simulink model "RCAM_simulation_trim_template"  (R2021b)
settings: Solver=VariableStepAuto  StartTime=0.0  StopTime=TF  RelTol=1e-3
values from neighbouring files (symbols this model uses):
  x0 = [75 ... (first row only)    [initializeConstants.m]
undefined symbols (not defined in the file or in its folder): RCAM_model
settings Model: Creator=khanh  LastModifiedBy=khanh

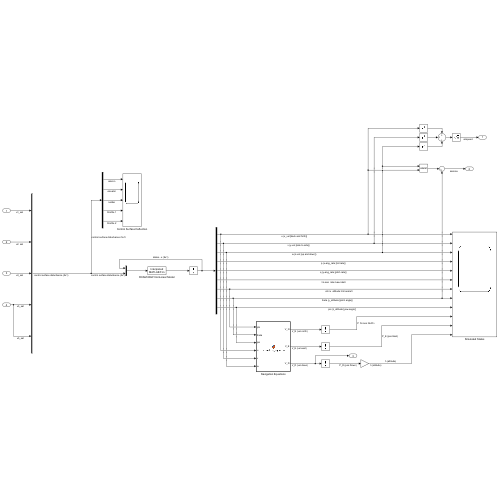
[thumbnail: Simulink's stored preview of the top-level diagram]
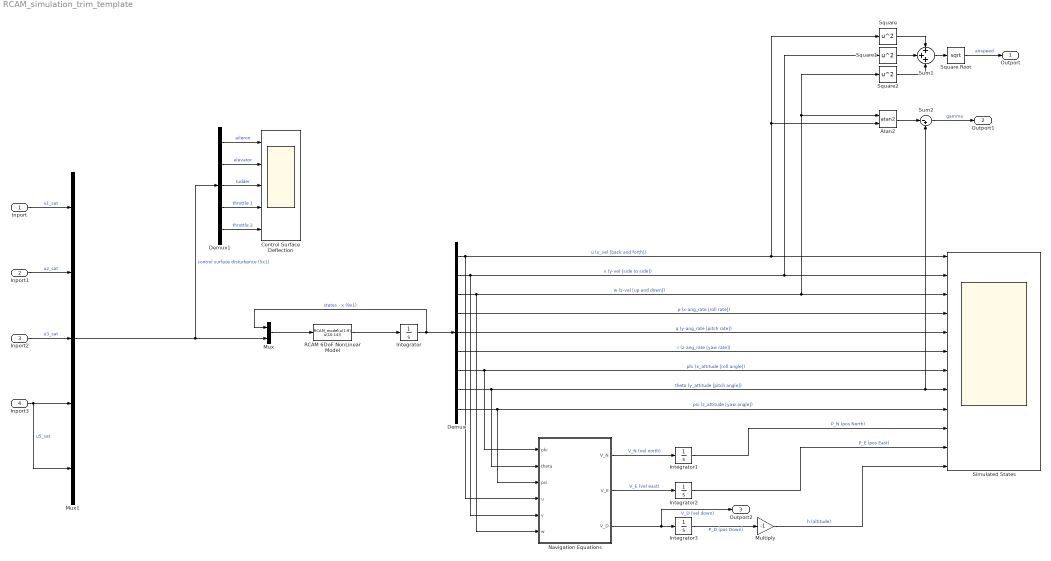
== system RCAM_simulation_trim_template ==
  Inport : Inport
  Inport1 : Inport  Port=2
  Inport2 : Inport  Port=3
  Inport3 : Inport  Port=4
  Atan2 : Trigonometry  Operator=atan2
  Control Surface Deflection : Scope  NumInputPorts=5
  Demux : Demux  Outputs=9
  Demux1 : Demux  Outputs=5
  Integrator : Integrator  InitialCondition=x0
  Integrator1 : Integrator  ContinuousStateAttributes='P_N'
  Integrator2 : Integrator  ContinuousStateAttributes='P_E'
  Integrator3 : Integrator  ContinuousStateAttributes='P_D'
  Multiply : Gain  Gain=-1
  Mux : Mux  Inputs=2
  Mux1 : Mux  Inputs=5
  Navigation Equations : MATLAB Function  TreatAsAtomicUnit=on
  RCAM 6DoF NonLinear Model : MATLABFcn  MATLABFcn=RCAM_model(u(1:9), u(10:14))
  Simulated States : Scope  NumInputPorts=12
  Square : Math  Operator=square  SaturateOnIntegerOverflow=on
  Square Root : Sqrt  SaturateOnIntegerOverflow=on
  Square1 : Math  Operator=square  SaturateOnIntegerOverflow=on
  Square2 : Math  Operator=square  SaturateOnIntegerOverflow=on
  Sum1 : Sum  Inputs=+++
  Sum2 : Sum  Inputs=|-+
  Outport : Outport
  Outport1 : Outport  Port=2
  Outport2 : Outport  Port=3
  wires:
  RCAM 6DoF NonLinear Model/1 -> Integrator/1
  Integrator/1 -> Demux/1, Mux/1  "states - x (9x1)"
  Mux/1 -> RCAM 6DoF NonLinear Model/1
  Inport/1 -> Mux1/1  "u1_sat"
  Inport3/1 -> Mux1/5, Mux1/4  "u5_sat"
  Inport2/1 -> Mux1/3  "u3_sat"
  Inport1/1 -> Mux1/2  "u2_sat"
  Demux1/1 -> Control Surface Deflection/1  "aileron"
  Demux1/2 -> Control Surface Deflection/2  "elevator"
  Demux1/3 -> Control Surface Deflection/3  "rudder"
  Demux1/4 -> Control Surface Deflection/4  "throttle 1"
  Demux1/5 -> Control Surface Deflection/5  "throttle 2"
  Mux1/1 -> Demux1/1, Mux/2  "control surface disturbance (5x1)"
  Demux/1 -> Navigation Equations/4(u), Atan2/2, Square/1, Simulated States/1  "u (x_vel [back and forth])"
  Demux/2 -> Navigation Equations/5(v), Square1/1, Simulated States/2  "v (y-vel [side to side])"
  Demux/3 -> Navigation Equations/6(w), Atan2/1, Square2/1, Simulated States/3  "w (z-vel [up and down])"
  Demux/4 -> Simulated States/4  "p (x-ang_rate [roll rate])"
  Demux/5 -> Simulated States/5  "q (y-ang_rate [pitch rate])"
  Demux/6 -> Simulated States/6  "r (z-ang_rate [yaw rate])"
  Demux/8 -> Navigation Equations/2(theta), Sum2/2, Simulated States/8  "theta (y_attitude [pitch angle])"
  Demux/9 -> Navigation Equations/3(psi), Simulated States/9  "psi (z_attitude [yaw angle])"
  Navigation Equations/3(V_D) -> Outport2/1, Integrator3/1  "V_D (vel down)"
  Navigation Equations/2(V_E) -> Integrator2/1  "V_E (vel east)"
  Navigation Equations/1(V_N) -> Integrator1/1  "V_N (vel north)"
  Integrator1/1 -> Simulated States/10  "P_N (pos North)"
  Integrator2/1 -> Simulated States/11  "P_E (pos East)"
  Integrator3/1 -> Multiply/1  "P_D (pos Down)"
  Demux/7 -> Navigation Equations/1(phi), Simulated States/7  "phi (x_attitude [roll angle])"
  Multiply/1 -> Simulated States/12  "h (altitude)"
  Square/1 -> Sum1/1
  Square1/1 -> Sum1/2
  Square2/1 -> Sum1/3
  Sum1/1 -> Square Root/1
  Square Root/1 -> Outport/1  "airspeed"
  Atan2/1 -> Sum2/1
  Sum2/1 -> Outport1/1  "gamma"

== matlab function RCAM_simulation_trim_template/Navigation Equations ==
  data: phi input; theta input; psi input; u input; V_N output; v input; w input; V_E output; V_D output
function [V_N, V_E, V_D] = navigation_equation(phi, theta, psi, u, v, w)

x7 = phi;
x8 = theta;
x9 = psi;
x1 = u;
x2 = v;
x3 = w;

V_b = [x1; x2; x3];

%navigation equations
C1v = [cos(x9) sin(x9) 0; -sin(x9) cos(x9) 0; 0 0 1];

C21 = [cos(x8) 0 -sin(x8); 0 1 0; sin(x8) 0 cos(x8)];

Cb2 = [1 0 0; 0 cos(x7) sin(x7); 0 -sin(x7) cos(x7)];

Cvb = Cb2*C21*C1v;
Cvb = Cvb';

vel_vector = Cvb*V_b;

V_N = vel_vector(1);
V_E = vel_vector(2);
V_D = vel_vector(3);

end
